simulink model "Colorspace_Conv"  (Simulink 6.4)
settings: Solver=ode45  StartTime=0.0  StopTime=10.0  RelTol=1e-3
undefined symbols (not defined in the file): jet, Rec, SDTV
libraries: vipconversions x4, vipsnks x2, vipsrcs x1
settings Model: LastModifiedBy=Pr . Saddam&Ali

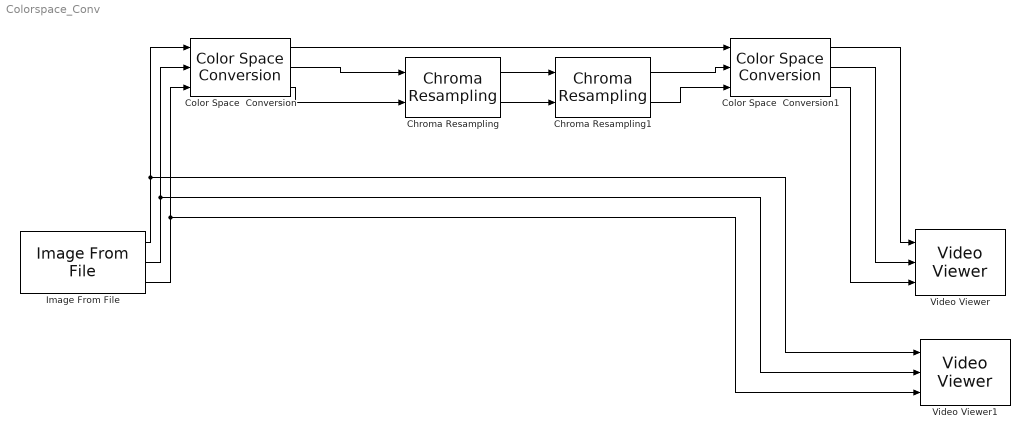
== system Colorspace_Conv ==
  Chroma Resampling : vipconversions/Chroma Resampling  resampling=4:4:4 to 4:2:2  interpolation=linear  antialiasing=Default  hcoeff=[0.2 0.6 0.2]  vcoeff=[0.5 0.5]
  Chroma Resampling1 : vipconversions/Chroma Resampling  resampling=4:2:2 to 4:4:4  interpolation=linear  antialiasing=Default  hcoeff=[0.2 0.6 0.2]  vcoeff=[0.5 0.5]
  Color Space  Conversion : vipconversions/Color Space  Conversion  conversion=R'G'B' to Y'CbCr  wp_str=D65  rec=Rec. 601 (SDTV)  sys=1125/60/2:1
  Color Space  Conversion1 : vipconversions/Color Space  Conversion  conversion=Y'CbCr to R'G'B'  wp_str=D65  rec=Rec. 601 (SDTV)  sys=1125/60/2:1
  Image From File : vipsrcs/Image From File  DialogController=vipDDGCreate  DialogControllerArgs=DataTag0  SystemSampleTime=-1  FileName=peppers.png  Ts=inf  ImageDataType=Inherit from input image  Signed=on  WordLength=16  sdImageDataType=uint(8)  FractionLengthMode=User-defined  FractionLength=15  OutPortLabels=R|G|B
  Video Viewer : vipsnks/Video Viewer  inputType=RGB  useColorMap=off  colormapValue=jet(256);  specRange=off  minInputVal=0  maxInputVal=255  FigPos=[256 264 512 384]  AxisZoom=on  trueSizedOnce=on
  Video Viewer1 : vipsnks/Video Viewer  inputType=RGB  useColorMap=off  colormapValue=jet(256);  specRange=off  minInputVal=0  maxInputVal=255  FigPos=[256 264 512 384]  AxisZoom=on  trueSizedOnce=on
  wires:
  Color Space  Conversion/1 -> Color Space  Conversion1/1
  Image From File/1 -> Color Space  Conversion/1, Video Viewer1/1
  Image From File/2 -> Color Space  Conversion/2, Video Viewer1/2
  Image From File/3 -> Color Space  Conversion/3, Video Viewer1/3
  Color Space  Conversion/2 -> Chroma Resampling/1
  Color Space  Conversion/3 -> Chroma Resampling/2
  Chroma Resampling/1 -> Chroma Resampling1/1
  Chroma Resampling/2 -> Chroma Resampling1/2
  Chroma Resampling1/1 -> Color Space  Conversion1/2
  Chroma Resampling1/2 -> Color Space  Conversion1/3
  Color Space  Conversion1/1 -> Video Viewer/1
  Color Space  Conversion1/2 -> Video Viewer/2
  Color Space  Conversion1/3 -> Video Viewer/3
